simulink model "multiplexer"  (R2017b)
settings: Solver=VariableStepAuto  StartTime=0.0  StopTime=10.0  RelTol=1e-3
settings Model: Creator=Ray  LastModifiedBy=Ray

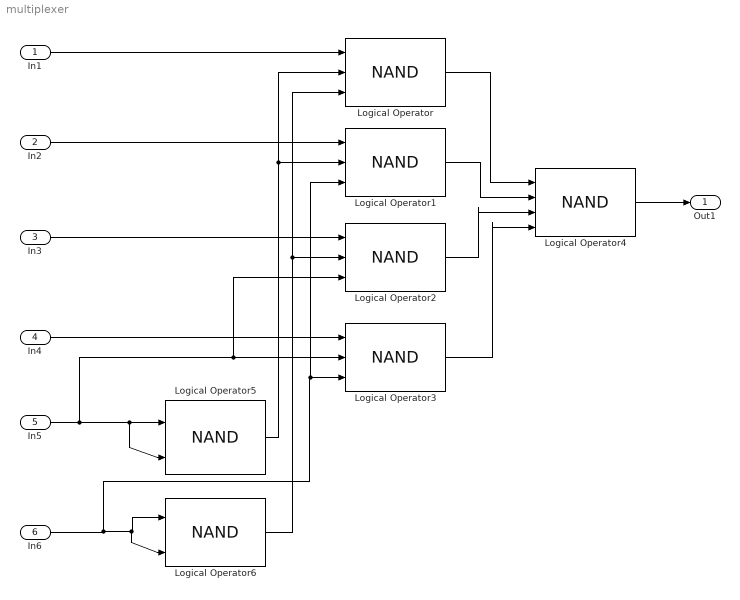
== system multiplexer ==
  In1 : Inport  OutDataTypeStr=boolean  SampleTime=1
  In2 : Inport  Port=2  OutDataTypeStr=boolean  SampleTime=1
  In3 : Inport  Port=3  OutDataTypeStr=boolean  SampleTime=1
  In4 : Inport  Port=4  OutDataTypeStr=boolean  SampleTime=1
  In5 : Inport  Port=5  OutDataTypeStr=boolean  SampleTime=1
  In6 : Inport  Port=6  OutDataTypeStr=boolean  SampleTime=1
  Logical Operator{,1..3} (4 alike) : Logic  Operator=NAND  Inputs=3  IconShape=distinctive  AllPortsSameDT=off  OutDataTypeStr=boolean
  Logical Operator4 : Logic  Operator=NAND  Inputs=4  IconShape=distinctive  AllPortsSameDT=off  OutDataTypeStr=boolean
  Logical Operator5 : Logic  Operator=NAND  IconShape=distinctive  AllPortsSameDT=off  OutDataTypeStr=boolean
  Logical Operator6 : Logic  Operator=NAND  IconShape=distinctive  AllPortsSameDT=off  OutDataTypeStr=boolean
  Out1 : Outport
  wires:
  In1/1 -> Logical Operator/1
  In2/1 -> Logical Operator1/1
  In3/1 -> Logical Operator2/1
  In4/1 -> Logical Operator3/1
  In5/1 -> Logical Operator5/2, Logical Operator5/1, Logical Operator2/3, Logical Operator3/2
  In6/1 -> Logical Operator6/2, Logical Operator6/1, Logical Operator1/3, Logical Operator3/3
  Logical Operator5/1 -> Logical Operator1/2, Logical Operator/2
  Logical Operator6/1 -> Logical Operator2/2, Logical Operator/3
  Logical Operator1/1 -> Logical Operator4/2
  Logical Operator2/1 -> Logical Operator4/3
  Logical Operator/1 -> Logical Operator4/1
  Logical Operator3/1 -> Logical Operator4/4
  Logical Operator4/1 -> Out1/1
